simulink model "VOO"  (R2020a)
settings: Solver=VariableStepAuto  StartTime=0.0  StopTime=10.0  RelTol=1e-3
settings Model: Creator=Costco Member  LastModifiedBy=Costco Member

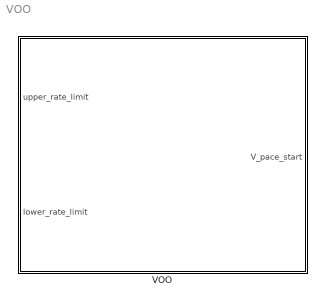
== system VOO ==
  VOO : Stateflow chart  TreatAsAtomicUnit=on

== stateflow chart VOO/VOO ==
  state Initial
    entry:
    V_pace_start=false;
  state Pace
    entry:
    V_pace_start=true;
    after(1,msec);
  (default) -> Initial
  Initial -> Pace : after(lower_rate_limit,msec)
  Pace -> Initial
  data: V_pace_start output boolean; upper_rate_limit input; lower_rate_limit input
